simulink model "passive_cell_balancing"  (R2022b)
settings: Solver=VariableStepAuto  StartTime=0.0  StopTime=600  RelTol=1e-3
undefined symbols (not defined in the file): Ion, Lithium
libraries: spsSeriesRLCBranchLib x4, spsBatteryLib x3, spsIGBTLib x3, spsIdealSwitchLib x2, spsDCVoltageSourceLib x1, sps_lib x1
settings Model: Creator=Aryan Aggarwal  LastModifiedBy=Aryan Aggarwal

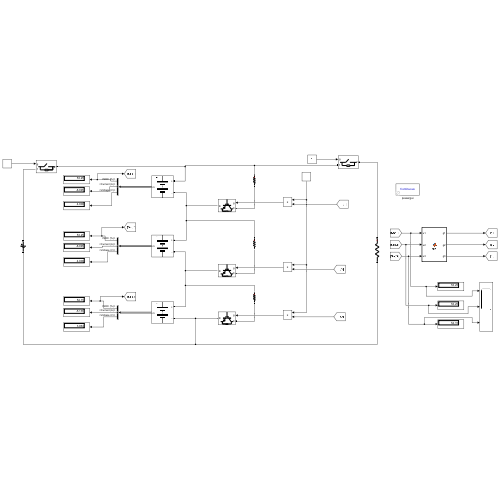
[thumbnail: Simulink's stored preview of the top-level diagram]
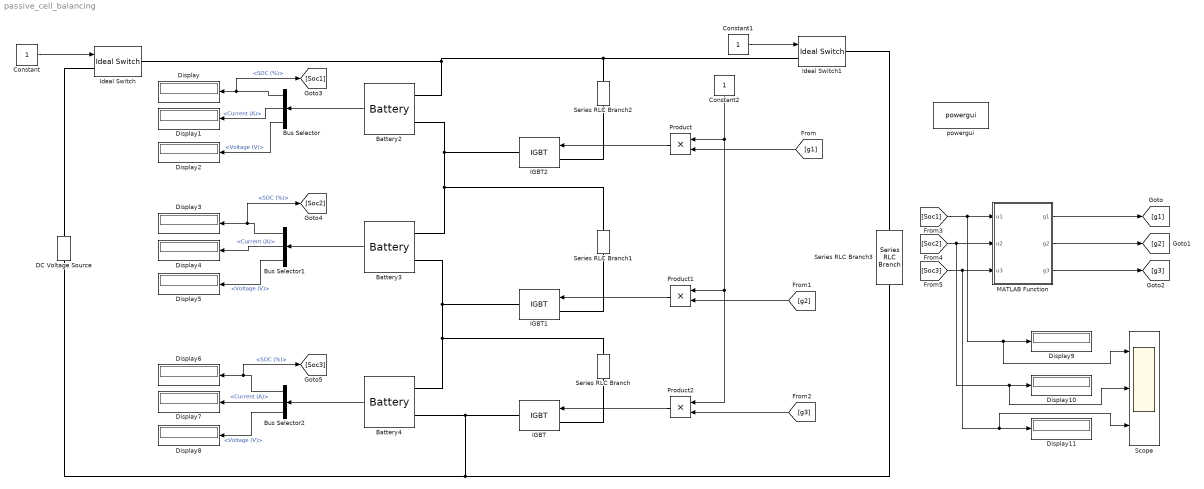
== system passive_cell_balancing ==
  Battery2 : spsBatteryLib/Battery  BatType=Lithium-Ion  ShowTempParam=off  ThermalPreset=no  ShowAgeParam=off  NomV=3.6  NomQ=5.4  SOC=20  Batt_Tr=30  PresetModel=on  MaxQ=5.4  MinV=2.7  FullV=4.1904  Dis_rate=2.3478  R=0.0066667  Normal_OP=4.8835  expZone="[3.8894      0.2653]"  current=[6.5 13 32.5]  Units=Time  Tci=20  NomT=20  T2=-30  MaxQ2=4.8  FullV2=7.1  Normal_OP2=5.655  expZone2="[6.58           1]"  Rca=0.6  ti=2000  Dp=0  Neq0=0  Tsim=1e6  Ta1=25  Qeol=5.4*0.9  Reol=0.013333*1.2  Char_age=[2.3478, 3]  Dis_age=[2.3478, 10]  N1=1500  N2=10500  N3=1000  N4=1400  Ta2=45  N5=950
  Battery3 : spsBatteryLib/Battery  BatType=Lithium-Ion  ShowTempParam=off  ThermalPreset=no  ShowAgeParam=off  NomV=3.6  NomQ=5.4  SOC=25  Batt_Tr=30  PresetModel=on  MaxQ=5.4  MinV=2.7  FullV=4.1904  Dis_rate=2.3478  R=0.0066667  Normal_OP=4.8835  expZone="[3.8894      0.2653]"  current=[6.5 13 32.5]  Units=Time  Tci=20  NomT=20  T2=-30  MaxQ2=4.8  FullV2=7.1  Normal_OP2=5.655  expZone2="[6.58           1]"  Rca=0.6  ti=2000  Dp=0  Neq0=0  Tsim=1e6  Ta1=25  Qeol=5.4*0.9  Reol=0.013333*1.2  Char_age=[2.3478, 3]  Dis_age=[2.3478, 10]  N1=1500  N2=10500  N3=1000  N4=1400  Ta2=45  N5=950
  Battery4 : spsBatteryLib/Battery  BatType=Lithium-Ion  ShowTempParam=off  ThermalPreset=no  ShowAgeParam=off  NomV=3.6  NomQ=5.4  SOC=30  Batt_Tr=30  PresetModel=on  MaxQ=5.4  MinV=2.7  FullV=4.1904  Dis_rate=2.3478  R=0.0066667  Normal_OP=4.8835  expZone="[3.8894      0.2653]"  current=[6.5 13 32.5]  Units=Time  Tci=20  NomT=20  T2=-30  MaxQ2=4.8  FullV2=7.1  Normal_OP2=5.655  expZone2="[6.58           1]"  Rca=0.6  ti=2000  Dp=0  Neq0=0  Tsim=1e6  Ta1=25  Qeol=5.4*0.9  Reol=0.013333*1.2  Char_age=[2.3478, 3]  Dis_age=[2.3478, 10]  N1=1500  N2=10500  N3=1000  N4=1400  Ta2=45  N5=950
  Bus Selector : BusSelector  OutputSignals=SOC (%),Current (A),Voltage (V)
  Bus Selector1 : BusSelector  OutputSignals=SOC (%),Current (A),Voltage (V)
  Bus Selector2 : BusSelector  OutputSignals=SOC (%),Current (A),Voltage (V)
  Constant : Constant
  Constant1 : Constant
  Constant2 : Constant
  DC Voltage Source : spsDCVoltageSourceLib/DC Voltage Source  Amplitude=12  Measurements=None
  Display{,1..11} (12 alike) : Display
  IGBT : spsIGBTLib/IGBT  Ron=0.001  Lon=0  Vf=1  Tf=1e-6  Tt=2e-6  IC=0  Rs=1e5  Cs=inf  Measurements=off
  IGBT1 : spsIGBTLib/IGBT  Ron=0.001  Lon=0  Vf=1  Tf=1e-6  Tt=2e-6  IC=0  Rs=1e5  Cs=inf  Measurements=off
  IGBT2 : spsIGBTLib/IGBT  Ron=0.001  Lon=0  Vf=1  Tf=1e-6  Tt=2e-6  IC=0  Rs=1e5  Cs=inf  Measurements=off
  Ideal Switch : spsIdealSwitchLib/Ideal Switch  Ron=0.001  Lon=0  IC=0  Rs=1e5  Cs=inf  Measurements=off
  Ideal Switch1 : spsIdealSwitchLib/Ideal Switch  Ron=0.001  Lon=0  IC=0  Rs=1e5  Cs=inf  Measurements=off
  MATLAB Function : MATLAB Function  TreatAsAtomicUnit=on
  Product : Product
  Product1 : Product
  Product2 : Product
  Scope : Scope  NumInputPorts=3
  Series RLC Branch{,1..3} (4 alike) : spsSeriesRLCBranchLib/Series RLC Branch  LConnTagsString=__new0  RConnTagsString=__new0  BranchType=R  Resistance=1  Inductance=1e-3  SetiL0=off  InitialCurrent=0  Capacitance=1e-6  Setx0=off  InitialVoltage=0  Measurements=None
  powergui : sps_lib/powergui  Priority=1  SimulationMode=Continuous  SampleTime=50e-6  frequency=60  Iterations=50  frequencyindice=0  Pbase=100e6  ErrMax=1e-4  UnitsV=kV  UnitsW=MW  buscounter=0  FunctionMessages=off  echomessages=off  EnableUseOfTLC=off  CurrentSourceSwitches=off  DisableSnubberDevices=off  DisableRonSwitches=off  DisableVfSwitches=off  DisplayEquations=off  AutomaticDiscreteSolvers=off  SolverType=Tustin/Backward Euler (TBE)  Interpol=off  ExternalGateDelay=off  methode=off  Ts=100  x0status=blocks  SPID=on  SwTol=0  HookPort=off  NonlinearTolerance=1e-4  nMaxIteration=100  ContinueOnMaxIteration=off  RestoreLinks=warning  ResistiveCurrentMeasurement=off  Frange=[0:2:500]  Ylog=off  Xlog=on  ShowGrid=off  save=off  variable=ZData  structure=0  ZoomFFT=off  StartTime=0.0  cycles=1  DisplayStyle=1  fundamental=60  FreqAxis=off  MaxFrequency=1000  frequencyindicesteady=1  RmsSteady=1  display=off
  wires:
  Constant/1 -> Ideal Switch/1
  Constant1/1 -> Ideal Switch1/1
  Battery2/1 -> Bus Selector/1
  Battery3/1 -> Bus Selector1/1
  Battery4/1 -> Bus Selector2/1
  Bus Selector/1 -> [Soc1], Display/1  "<SOC (%)>"
  Bus Selector/2 -> Display1/1  "<Current (A)>"
  Bus Selector/3 -> Display2/1  "<Voltage (V)>"
  Bus Selector1/1 -> [Soc2], Display3/1  "<SOC (%)>"
  Bus Selector1/2 -> Display4/1  "<Current (A)>"
  Bus Selector1/3 -> Display5/1  "<Voltage (V)>"
  Bus Selector2/1 -> [Soc3], Display6/1  "<SOC (%)>"
  Bus Selector2/2 -> Display7/1  "<Current (A)>"
  Bus Selector2/3 -> Display8/1  "<Voltage (V)>"
  Constant2/1 -> Product2/1, Product1/1, Product/1
  [g1] -> Product/2
  [g2] -> Product1/2
  [g3] -> Product2/2
  Product/1 -> IGBT2/1
  Product1/1 -> IGBT1/1
  Product2/1 -> IGBT/1
  MATLAB Function/1(g1) -> [g1]
  MATLAB Function/3(g3) -> [g3]
  MATLAB Function/2(g2) -> [g2]
  [Soc1] -> Scope/1, Display9/1, MATLAB Function/1(u1)
  [Soc2] -> Scope/2, Display10/1, MATLAB Function/2(u2)
  [Soc3] -> Scope/3, Display11/1, MATLAB Function/3(u3)
  connections:
  Battery2/LConn2 -- IGBT2/RConn1 -- Series RLC Branch1/LConn1 -- Battery3/LConn1
  Battery3/LConn2 -- IGBT1/RConn1 -- Battery4/LConn1 -- Series RLC Branch/LConn1
  Series RLC Branch/RConn1 -- IGBT/LConn1
  IGBT1/LConn1 -- Series RLC Branch1/RConn1
  IGBT2/LConn1 -- Series RLC Branch2/RConn1
  Series RLC Branch2/LConn1 -- Ideal Switch1/LConn1 -- Ideal Switch/RConn1 -- Battery2/LConn1
  Series RLC Branch3/LConn1 -- Ideal Switch1/RConn1
  DC Voltage Source/RConn1 -- Ideal Switch/LConn1
  IGBT/RConn1 -- Series RLC Branch3/RConn1 -- DC Voltage Source/LConn1 -- Battery4/LConn2

== matlab function passive_cell_balancing/MATLAB Function ==
  data: u1 input; g1 output; u2 input; u3 input; g2 output; g3 output
function [g1,g2,g3] = fcn(u1,u2,u3)

u1 = u1*1000;
u2 = u2*1000;
u3 = u3 *1000;


u1= int32(u1);
u2= int32(u2);
u3= int32(u3);

if u1>u2||u1>u3
    g1=1
else
    g1=0
end

if u2>u1||u2>u3
    g2=1
else
    g2=0
end

if u3>u1||u3>u2
    g3=1
else
    g3=0
end
end
